simulink model "Que_6"  (R2020b)
settings: Solver=VariableStepAuto  StartTime=0.0  StopTime=10  RelTol=1e-3
settings Model: Creator=hp  LastModifiedBy=hp

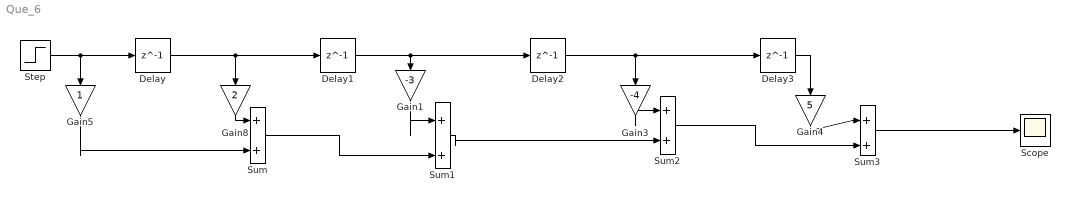
== system Que_6 ==
  Delay{,1..3} (4 alike) : Delay  DelayLength=1  InitialCondition=0
  Gain1 : Gain  Gain=-3
  Gain3 : Gain  Gain=-4
  Gain4 : Gain  Gain=5
  Gain5 : Gain
  Gain8 : Gain  Gain=2
  Scope : Scope
  Step : Step  SampleTime=0
  Sum{,1..3} (4 alike) : Sum  Inputs=|++
  wires:
  Step/1 -> Gain5/1, Delay/1
  Gain5/1 -> Sum/2
  Delay/1 -> Delay1/1, Gain8/1
  Gain8/1 -> Sum/1
  Sum/1 -> Sum1/2
  Delay1/1 -> Delay2/1, Gain1/1
  Gain1/1 -> Sum1/1
  Sum1/1 -> Sum2/2
  Gain3/1 -> Sum2/1
  Delay2/1 -> Delay3/1, Gain3/1
  Sum2/1 -> Sum3/2
  Delay3/1 -> Gain4/1
  Gain4/1 -> Sum3/1
  Sum3/1 -> Scope/1
